simulink model "speakermodel"  (R2015b)
settings: Solver=ode4  StartTime=0.0  StopTime=0.02  FixedStep=0.00001  RelTol=1e-3
values from neighbouring files (symbols this model uses):
  b = 50    [parameters.m]
  k = 2E5    (= 200000)    [parameters.m]
  Kf = 2*pi*r*N*beta    (= 3.14159265359)    [parameters.m]
  L = 0.05E-3    (= 5e-05)    [parameters.m]
  m = 4E-3    (= 0.004)    [parameters.m]
  R = 5    [parameters.m]
settings Model: ExtModeTrigDuration=10000  Creator=millerid  LastModifiedBy=millerid
settings SolverCC: PositivePriorityOrder=on
settings RTWCC: SystemTargetFile=quarc_win64.tlc  TemplateMakefile=quarc_default_tmf  Description=QUARC Win64 Target
settings STFCustomTargetCC: TargetPreCompLibLocation=C:\ProgramData\QUARC\lib\2015b\win64\release  GeneratePreprocessorConditionals=Use local settings  CPPClassGenCompliant=off
settings GRTTargetCC: TargetPreCompLibLocation=C:\ProgramData\QUARC\lib\2015b\win64\release  ParMdlRefBuildCompliant=off  CompOptLevelCompliant=off  CombineOutputUpdateFcns=off  MatFileLogging=off  CPPClassGenCompliant=off  GRTInterface=on  UseToolchainInfoCompliant=off  ExtMode=on  ExtModeMexFile=quarc_comm

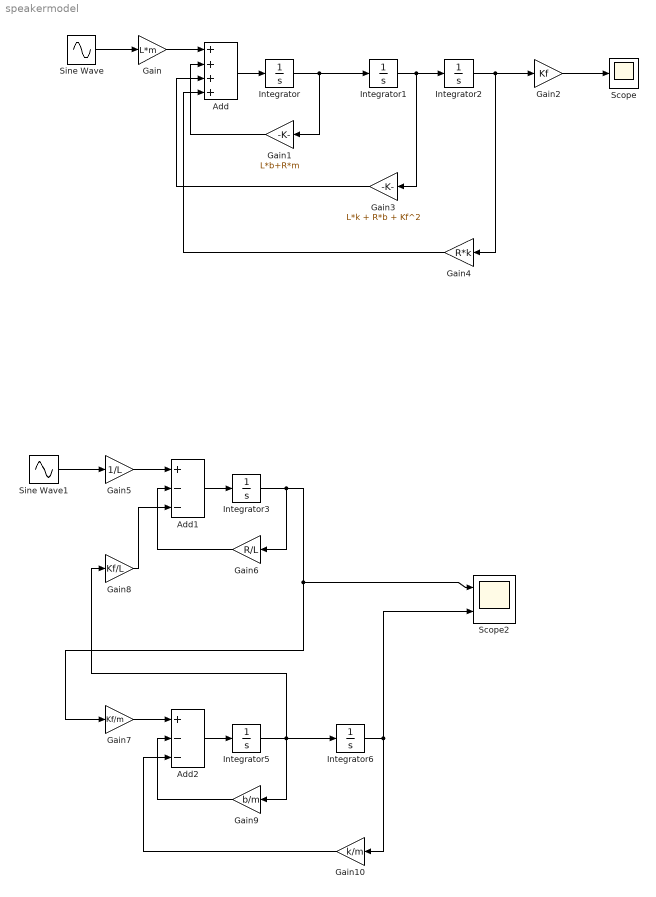
== system speakermodel ==
  Add : Sum  Inputs=++++
  Add1 : Sum  Inputs=+--
  Add2 : Sum  Inputs=+--
  Gain : Gain  Gain=L*m
  Gain1 : Gain  Gain=L*b+R*m
  Gain10 : Gain  Gain=k/m
  Gain2 : Gain  Gain=Kf
  Gain3 : Gain  Gain=L*k + R*b + Kf^2
  Gain4 : Gain  Gain=R*k
  Gain5 : Gain  Gain=1/L
  Gain6 : Gain  Gain=R/L
  Gain7 : Gain  Gain=Kf/m
  Gain8 : Gain  Gain=Kf/L
  Gain9 : Gain  Gain=b/m
  Integrator{,1..3,5..6} (6 alike) : Integrator
  Scope : Scope
  Scope2 : Scope  NumInputPorts=2
  Sine Wave : Sin  Frequency=200  SampleTime=0
  Sine Wave1 : Sin  Frequency=20000  SampleTime=0
  wires:
  Integrator/1 -> Gain1/1, Integrator1/1
  Integrator1/1 -> Gain3/1, Integrator2/1
  Sine Wave/1 -> Gain/1
  Gain/1 -> Add/1
  Add/1 -> Integrator/1
  Gain1/1 -> Add/2
  Integrator2/1 -> Gain2/1, Gain4/1
  Gain3/1 -> Add/3
  Gain4/1 -> Add/4
  Gain2/1 -> Scope/1
  Integrator3/1 -> Gain6/1, Scope2/1, Gain7/1
  Add1/1 -> Integrator3/1
  Gain6/1 -> Add1/2
  Integrator5/1 -> Gain9/1, Gain8/1, Integrator6/1
  Gain7/1 -> Add2/1
  Add2/1 -> Integrator5/1
  Gain9/1 -> Add2/2
  Gain10/1 -> Add2/3
  Integrator6/1 -> Scope2/2, Gain10/1
  Sine Wave1/1 -> Gain5/1
  Gain5/1 -> Add1/1
  Gain8/1 -> Add1/3
